simulink model "phaseDelay"  (R2015a)
settings: Solver=ode45  StartTime=0.0  StopTime=10.0  RelTol=1e-3
settings Model: Creator=John  LastModifiedBy=John

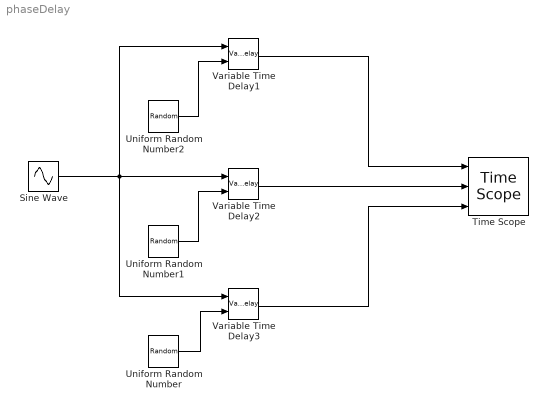
== system phaseDelay ==
  Sine Wave : Sin  Frequency=2*pi*[10 20 30]*1e6  SampleTime=0
  Time Scope : TimeScope  DefaultConfigurationName=spbscopes.TimeScopeBlockCfg  NumInputPorts=3
  Uniform Random Number : UniformRandomNumber  SampleTime=0.1
  Uniform Random Number1 : UniformRandomNumber  SampleTime=0.1
  Uniform Random Number2 : UniformRandomNumber  SampleTime=0.1
  Variable Time Delay1 : VariableTransportDelay  MaximumDelay=10
  Variable Time Delay2 : VariableTransportDelay  MaximumDelay=10
  Variable Time Delay3 : VariableTransportDelay  MaximumDelay=10
  wires:
  Sine Wave/1 -> Variable Time Delay3/1, Variable Time Delay2/1, Variable Time Delay1/1
  Variable Time Delay2/1 -> Time Scope/2
  Variable Time Delay3/1 -> Time Scope/3
  Uniform Random Number/1 -> Variable Time Delay3/2
  Uniform Random Number1/1 -> Variable Time Delay2/2
  Uniform Random Number2/1 -> Variable Time Delay1/2
  Variable Time Delay1/1 -> Time Scope/1
